simulink model "blockdemo"  (Simulink 6.3)
settings: Solver=FixedStepDiscrete  StartTime=0  StopTime=20  FixedStep=1  RelTol=1e-3
InitFcn:
  | %% DSPBuilder Start
  | alt_dspbuilder_update_model(bdroot)
  | %% DSPBuilder End
libraries: allblocks_alteradspbuilder2 x5
settings Model: Creator=mjervis  LastModifiedBy=delphick

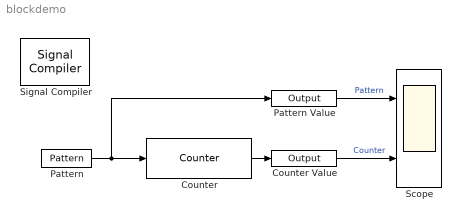
== system blockdemo ==
  Counter : allblocks_alteradspbuilder2/Counter  BusType=Unsigned Integer  bwl=8  bwr=0  use_modulo=on  modulo=256  SpecifyClock=off  direction=Increment  use_sload=off  use_sset=off  svalue=1  use_ena=on  use_sclr=off
  Counter Value : allblocks_alteradspbuilder2/Output  iofile=C:\workspace_clean\Documentation\DesignExamples\Tutorials\UnitBlocks\GateAndControl\Pattern\tb_blockdemo\blockdemo_Counter+Value.capture  BusType=Unsigned Integer  bwl=8  bwr=0  PORTTYPE=Output
  Pattern : allblocks_alteradspbuilder2/Pattern  Sequence=100  SpecifyClock=off  use_ena=off  use_sclr=off
  Pattern Value : allblocks_alteradspbuilder2/Output  iofile=C:\workspace_clean\Documentation\DesignExamples\Tutorials\UnitBlocks\GateAndControl\Pattern\tb_blockdemo\blockdemo_Pattern+Value.capture  BusType=Single Bit  bwl=8  bwr=0  PORTTYPE=Output
  Scope : Scope  NumInputPorts=2
      settings: TimeRange=20  YMin=-2~0  YMax=2~10
  Signal Compiler : allblocks_alteradspbuilder2/Signal Compiler  DeviceFamily=Stratix IV  DeviceName=AUTO  EnableSignalTap=off  SignalTapDepth=128  UseBoardBlock=off  StpUseDefaultClock=on  StpClock=clock
  wires:
  Pattern/1 -> Counter/1, Pattern Value/1
  Counter/1 -> Counter Value/1
  Pattern Value/1 -> Scope/1  "Pattern"
  Counter Value/1 -> Scope/2  "Counter"
